simulink model "Q2c"  (R2021b)
settings: Solver=VariableStepAuto  StartTime=0.0  StopTime=16  RelTol=1e-3
undefined symbols (not defined in the file or in its folder): sigbuilder_block
libraries: simulink_extras x1
settings Model: Creator=adamj  LastModifiedBy=adamj

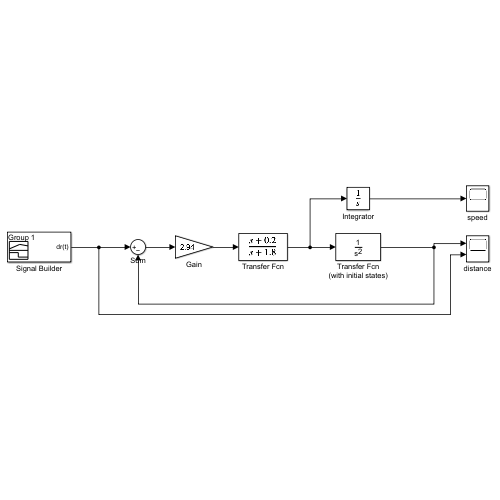
[thumbnail: Simulink's stored preview of the top-level diagram]
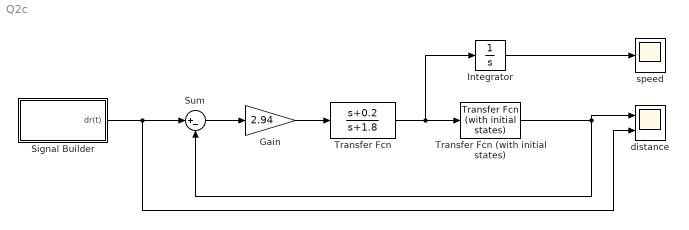
== system Q2c ==
  Gain : Gain  Gain=2.94
  Integrator : Integrator
  Signal Builder : Subsystem  Tag=STV Subsys  LoadFcn=sigbuilder_block('load');  StartFcn=sigbuilder_block('start');  StopFcn=sigbuilder_block('stop');  ClipboardFcn=sigbuilder_block('clipboard');  mask(Sigbuilder block){tuvar=[0:10]}
      mask help: Simulink:masks:SigbuilderBlock_MD
      mask init:
      | if ~strcmp(get_param(bdroot(gcbh),'SimulationStatus'),'stopped') tuvar = sigbuilder_block('maskInit'); end
      settings: CopyFcn=sigbuilder_block('copy');  DeleteFcn=sigbuilder_block('delete');  ModelCloseFcn=sigbuilder_block('modelClose');  PreSaveFcn=sigbuilder_block('preSave');  PauseFcn=sigbuilder_block('pause');  ContinueFcn=sigbuilder_block('continue');  NameChangeFcn=sigbuilder_block('namechange');  OpenFcn=sigbuilder_block('open',[10.2 166.8 555.6 244.2 ]);  CloseFcn=sigbuilder_block('close');
      mask Display: plot(0, 0, 100, 100,[2, 2, 32, 32, 2], [68, 8, 8, 68, 68],[32, 2], [38, 38], [32, 19, 2],[53, 60, 44], [32, 17, 17, 2],[16, 16, 31, 31]);txt = getActiveGroup(gcbh);text(2, 100, txt,'verticalAlignment', 'top');
  Sum : Sum  Inputs=|+-
  Transfer Fcn : TransferFcn  Numerator=[1 0.2]  Denominator=[1 1.8]
  Transfer Fcn (with initial states) : simulink_extras/Additional Linear/Transfer Fcn (with initial states)  N=[0 1]  D="[1 0  0]"  X0=1
  distance : Scope  NumInputPorts=2
  speed : Scope
  wires:
  Transfer Fcn (with initial states)/1 -> Sum/2, distance/1
  Transfer Fcn/1 -> Integrator/1, Transfer Fcn (with initial states)/1
  Signal Builder/1(dr(t)) -> distance/2, Sum/1
  Sum/1 -> Gain/1
  Gain/1 -> Transfer Fcn/1
  Integrator/1 -> speed/1

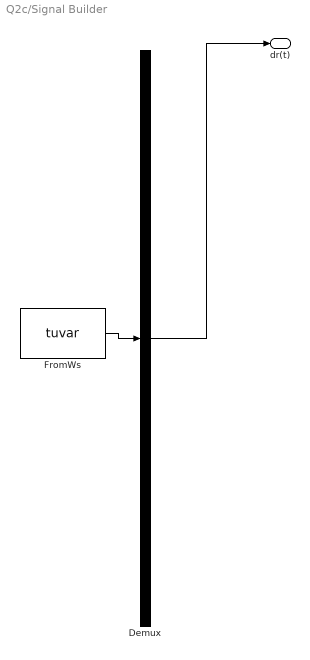
== system Q2c/Signal Builder ==
  Demux : Demux  Tag=STV Demux  Outputs=1
      settings: DisplayOption=none
  FromWs : FromWorkspace  Tag=STV FromWs  VariableName=tuvar
      SigBuilderData=|
      | common.afterFinalStr = 'Extrapolate'
      | common.sampleTime = 0
      | dataSet.timeRange = [0 50]
      | dataSet.name = 'Group 1'
      | sbobj.Groups.Name = 'Group 1'
      | sbobj.Groups.Signals.Name = 'dr(t)'
      | sbobj.Groups.Signals.XData = [0 4 8 50]
      | sbobj.Groups.Signals.YData = [1.5 1.5 0.7 0.7]
      | sbobj.Groups.TimeRange = [0 50]
  dr(t) : Outport  Tag=STV Outport
  wires:
  FromWs/1 -> Demux/1
  Demux/1 -> dr(t)/1
